simulink model "EHB_speedgoat_R2020a_V1"  (R2020a)
settings: Solver=FixedStepDiscrete  StartTime=0.0  StopTime=inf  FixedStep=0.001  RelTol=1e-3  EnableMultiTasking=on
model workspace (MAT data in the model file):
  A : Simulink.Signal (value not decoded)
  B : Simulink.Signal (value not decoded)
  C : Simulink.Signal (value not decoded)
  D : Simulink.Signal (value not decoded)
  E : Simulink.Signal (value not decoded)
  calin = [-9.96 -7.98 -5.98 -3.99 -1.994 0 1.995 3.992 5.99 7.98 9.97]
  calout = [-10 -8 -6 -4 -2 0 2 4 6 8 10]
symbols that are objects in the model workspace (value not decoded): C, D
undefined symbols (not defined in the file): Com1, none, ts_IO612
libraries: simulink x1436, xpcethercatlib x1223, yisutbxlib_utilities x256, xpcutilitieslib x156, hdlsllib x145, canmsglib x46, speedgoatlib_IO602_4 x11, speedgoatlib_IO611 x7, slrttcplib x4, CanManageLib x3, slrtlib x3, xpcseriallib x2
(part 11 of 30)

== system EHB_speedgoat_R2020a_V1/保留/TIF_01/YS4020_M_2/YS4020_M/FIU_CH13 ==
  FIU_SetCH2 : Inport
  "Bit Unpacking " : xpcutilitieslib/Bit Unpacking   SignExtend=on  MaskBitPatterns={[0],[1],[2],[3]}  MaskPackDataType=uint8  MaskPackDataSize=[1]  MaskUnpackDataTypes={'boolean','boolean','boolean','boolean'}  MaskUnpackDataSizes={[1],[1],[1],[1]}
      settings: SourceProductBaseCode=XP
  Bus Creator : BusCreator  Inputs=4
  Protect : Subsystem
  CH2_Out : Outport
  wires:
  Bus Creator/1 -> CH2_Out/1
  "Bit Unpacking "/4 -> Protect/4(Open_In)
  "Bit Unpacking "/3 -> Protect/3(COM_In)
  "Bit Unpacking "/2 -> Protect/2(KL31_In)
  "Bit Unpacking "/1 -> Protect/1(KL30_In)
  Protect/4(Open_Out) -> Bus Creator/4  "Open_Out"
  Protect/1(KL30_Out) -> Bus Creator/1  "KL30_Out"
  Protect/2(KL31_Out) -> Bus Creator/2  "KL31_Out"
  Protect/3(COM_Out) -> Bus Creator/3  "COM_Out"
  FIU_SetCH2/1 -> "Bit Unpacking "/1

== system EHB_speedgoat_R2020a_V1/保留/TIF_01/YS4020_M_2/YS4020_M/FIU_CH14 ==
  FIU_SetCH3 : Inport
  "Bit Unpacking " : xpcutilitieslib/Bit Unpacking   SignExtend=on  MaskBitPatterns={[0],[1],[2],[3]}  MaskPackDataType=uint8  MaskPackDataSize=[1]  MaskUnpackDataTypes={'boolean','boolean','boolean','boolean'}  MaskUnpackDataSizes={[1],[1],[1],[1]}
      settings: SourceProductBaseCode=XP
  Bus Creator : BusCreator  Inputs=4
  Protect : Subsystem
  CH3_Out : Outport
  wires:
  FIU_SetCH3/1 -> "Bit Unpacking "/1
  Protect/3(COM_Out) -> Bus Creator/3  "COM_Out"
  Protect/2(KL31_Out) -> Bus Creator/2  "KL31_Out"
  Protect/1(KL30_Out) -> Bus Creator/1  "KL30_Out"
  Protect/4(Open_Out) -> Bus Creator/4  "Open_Out"
  "Bit Unpacking "/1 -> Protect/1(KL30_In)
  "Bit Unpacking "/2 -> Protect/2(KL31_In)
  "Bit Unpacking "/3 -> Protect/3(COM_In)
  "Bit Unpacking "/4 -> Protect/4(Open_In)
  Bus Creator/1 -> CH3_Out/1

== system EHB_speedgoat_R2020a_V1/保留/TIF_01/YS4020_M_2/YS4020_M/FIU_CH15 ==
  FIU_SetCH4 : Inport
  "Bit Unpacking " : xpcutilitieslib/Bit Unpacking   SignExtend=on  MaskBitPatterns={[0],[1],[2],[3]}  MaskPackDataType=uint8  MaskPackDataSize=[1]  MaskUnpackDataTypes={'boolean','boolean','boolean','boolean'}  MaskUnpackDataSizes={[1],[1],[1],[1]}
      settings: SourceProductBaseCode=XP
  Bus Creator : BusCreator  Inputs=4
  Protect : Subsystem
  CH4_Out : Outport
  wires:
  Bus Creator/1 -> CH4_Out/1
  "Bit Unpacking "/4 -> Protect/4(Open_In)
  "Bit Unpacking "/3 -> Protect/3(COM_In)
  "Bit Unpacking "/2 -> Protect/2(KL31_In)
  "Bit Unpacking "/1 -> Protect/1(KL30_In)
  Protect/4(Open_Out) -> Bus Creator/4  "Open_Out"
  Protect/1(KL30_Out) -> Bus Creator/1  "KL30_Out"
  Protect/2(KL31_Out) -> Bus Creator/2  "KL31_Out"
  Protect/3(COM_Out) -> Bus Creator/3  "COM_Out"
  FIU_SetCH4/1 -> "Bit Unpacking "/1

== system EHB_speedgoat_R2020a_V1/保留/TIF_01/YS4020_M_2/YS4020_M/FIU_CH16 ==
  FIU_SetCH5 : Inport
  "Bit Unpacking " : xpcutilitieslib/Bit Unpacking   SignExtend=on  MaskBitPatterns={[0],[1],[2],[3]}  MaskPackDataType=uint8  MaskPackDataSize=[1]  MaskUnpackDataTypes={'boolean','boolean','boolean','boolean'}  MaskUnpackDataSizes={[1],[1],[1],[1]}
      settings: SourceProductBaseCode=XP
  Bus Creator : BusCreator  Inputs=4
  Protect : Subsystem
  CH5_Out : Outport
  wires:
  FIU_SetCH5/1 -> "Bit Unpacking "/1
  Protect/3(COM_Out) -> Bus Creator/3  "COM_Out"
  Protect/2(KL31_Out) -> Bus Creator/2  "KL31_Out"
  Protect/1(KL30_Out) -> Bus Creator/1  "KL30_Out"
  Protect/4(Open_Out) -> Bus Creator/4  "Open_Out"
  "Bit Unpacking "/1 -> Protect/1(KL30_In)
  "Bit Unpacking "/2 -> Protect/2(KL31_In)
  "Bit Unpacking "/3 -> Protect/3(COM_In)
  "Bit Unpacking "/4 -> Protect/4(Open_In)
  Bus Creator/1 -> CH5_Out/1

== system EHB_speedgoat_R2020a_V1/保留/TIF_01/YS4020_M_2/YS4020_M/FIU_CH17 ==
  FIU_SetCH6 : Inport
  "Bit Unpacking " : xpcutilitieslib/Bit Unpacking   SignExtend=on  MaskBitPatterns={[0],[1],[2],[3]}  MaskPackDataType=uint8  MaskPackDataSize=[1]  MaskUnpackDataTypes={'boolean','boolean','boolean','boolean'}  MaskUnpackDataSizes={[1],[1],[1],[1]}
      settings: SourceProductBaseCode=XP
  Bus Creator : BusCreator  Inputs=4
  Protect : Subsystem
  CH6_Out : Outport
  wires:
  Bus Creator/1 -> CH6_Out/1
  "Bit Unpacking "/4 -> Protect/4(Open_In)
  "Bit Unpacking "/3 -> Protect/3(COM_In)
  "Bit Unpacking "/2 -> Protect/2(KL31_In)
  "Bit Unpacking "/1 -> Protect/1(KL30_In)
  Protect/4(Open_Out) -> Bus Creator/4  "Open_Out"
  Protect/1(KL30_Out) -> Bus Creator/1  "KL30_Out"
  Protect/2(KL31_Out) -> Bus Creator/2  "KL31_Out"
  Protect/3(COM_Out) -> Bus Creator/3  "COM_Out"
  FIU_SetCH6/1 -> "Bit Unpacking "/1

== system EHB_speedgoat_R2020a_V1/保留/TIF_01/YS4020_M_2/YS4020_M/FIU_CH18 ==
  FIU_SetCH7 : Inport
  "Bit Unpacking " : xpcutilitieslib/Bit Unpacking   SignExtend=on  MaskBitPatterns={[0],[1],[2],[3]}  MaskPackDataType=uint8  MaskPackDataSize=[1]  MaskUnpackDataTypes={'boolean','boolean','boolean','boolean'}  MaskUnpackDataSizes={[1],[1],[1],[1]}
      settings: SourceProductBaseCode=XP
  Bus Creator : BusCreator  Inputs=4
  Protect : Subsystem
  CH7_Out : Outport
  wires:
  FIU_SetCH7/1 -> "Bit Unpacking "/1
  Protect/3(COM_Out) -> Bus Creator/3  "COM_Out"
  Protect/2(KL31_Out) -> Bus Creator/2  "KL31_Out"
  Protect/1(KL30_Out) -> Bus Creator/1  "KL30_Out"
  Protect/4(Open_Out) -> Bus Creator/4  "Open_Out"
  "Bit Unpacking "/1 -> Protect/1(KL30_In)
  "Bit Unpacking "/2 -> Protect/2(KL31_In)
  "Bit Unpacking "/3 -> Protect/3(COM_In)
  "Bit Unpacking "/4 -> Protect/4(Open_In)
  Bus Creator/1 -> CH7_Out/1

== system EHB_speedgoat_R2020a_V1/保留/TIF_01/YS4020_M_2/YS4020_M/FIU_CH19 ==
  FIU_SetCH8 : Inport
  "Bit Unpacking " : xpcutilitieslib/Bit Unpacking   SignExtend=on  MaskBitPatterns={[0],[1],[2],[3]}  MaskPackDataType=uint8  MaskPackDataSize=[1]  MaskUnpackDataTypes={'boolean','boolean','boolean','boolean'}  MaskUnpackDataSizes={[1],[1],[1],[1]}
      settings: SourceProductBaseCode=XP
  Bus Creator : BusCreator  Inputs=4
  Protect : Subsystem
  CH8_Out : Outport
  wires:
  Bus Creator/1 -> CH8_Out/1
  "Bit Unpacking "/4 -> Protect/4(Open_In)
  "Bit Unpacking "/3 -> Protect/3(COM_In)
  "Bit Unpacking "/2 -> Protect/2(KL31_In)
  "Bit Unpacking "/1 -> Protect/1(KL30_In)
  Protect/4(Open_Out) -> Bus Creator/4  "Open_Out"
  Protect/1(KL30_Out) -> Bus Creator/1  "KL30_Out"
  Protect/2(KL31_Out) -> Bus Creator/2  "KL31_Out"
  Protect/3(COM_Out) -> Bus Creator/3  "COM_Out"
  FIU_SetCH8/1 -> "Bit Unpacking "/1

== system EHB_speedgoat_R2020a_V1/保留/TIF_01/YS4020_M_2/YS4020_M/FIU_CH2 ==
  FIU_SetCH2 : Inport
  "Bit Unpacking " : xpcutilitieslib/Bit Unpacking   SignExtend=on  MaskBitPatterns={[0],[1],[2],[3]}  MaskPackDataType=uint8  MaskPackDataSize=[1]  MaskUnpackDataTypes={'boolean','boolean','boolean','boolean'}  MaskUnpackDataSizes={[1],[1],[1],[1]}
      settings: SourceProductBaseCode=XP
  Bus Creator : BusCreator  Inputs=4
  Protect : Subsystem
  CH2_Out : Outport
  wires:
  FIU_SetCH2/1 -> "Bit Unpacking "/1
  Protect/3(COM_Out) -> Bus Creator/3  "COM_Out"
  Protect/2(KL31_Out) -> Bus Creator/2  "KL31_Out"
  Protect/1(KL30_Out) -> Bus Creator/1  "KL30_Out"
  Protect/4(Open_Out) -> Bus Creator/4  "Open_Out"
  "Bit Unpacking "/1 -> Protect/1(KL30_In)
  "Bit Unpacking "/2 -> Protect/2(KL31_In)
  "Bit Unpacking "/3 -> Protect/3(COM_In)
  "Bit Unpacking "/4 -> Protect/4(Open_In)
  Bus Creator/1 -> CH2_Out/1

== system EHB_speedgoat_R2020a_V1/保留/TIF_01/YS4020_M_2/YS4020_M/FIU_CH20 ==
  FIU_SetCH9 : Inport
  "Bit Unpacking " : xpcutilitieslib/Bit Unpacking   SignExtend=on  MaskBitPatterns={[0],[1],[2],[3]}  MaskPackDataType=uint8  MaskPackDataSize=[1]  MaskUnpackDataTypes={'boolean','boolean','boolean','boolean'}  MaskUnpackDataSizes={[1],[1],[1],[1]}
      settings: SourceProductBaseCode=XP
  Bus Creator : BusCreator  Inputs=4
  Protect : Subsystem
  CH9_Out : Outport
  wires:
  FIU_SetCH9/1 -> "Bit Unpacking "/1
  Protect/3(COM_Out) -> Bus Creator/3  "COM_Out"
  Protect/2(KL31_Out) -> Bus Creator/2  "KL31_Out"
  Protect/1(KL30_Out) -> Bus Creator/1  "KL30_Out"
  Protect/4(Open_Out) -> Bus Creator/4  "Open_Out"
  "Bit Unpacking "/1 -> Protect/1(KL30_In)
  "Bit Unpacking "/2 -> Protect/2(KL31_In)
  "Bit Unpacking "/3 -> Protect/3(COM_In)
  "Bit Unpacking "/4 -> Protect/4(Open_In)
  Bus Creator/1 -> CH9_Out/1

== system EHB_speedgoat_R2020a_V1/保留/TIF_01/YS4020_M_2/YS4020_M/FIU_CH3 ==
  FIU_SetCH3 : Inport
  "Bit Unpacking " : xpcutilitieslib/Bit Unpacking   SignExtend=on  MaskBitPatterns={[0],[1],[2],[3]}  MaskPackDataType=uint8  MaskPackDataSize=[1]  MaskUnpackDataTypes={'boolean','boolean','boolean','boolean'}  MaskUnpackDataSizes={[1],[1],[1],[1]}
      settings: SourceProductBaseCode=XP
  Bus Creator : BusCreator  Inputs=4
  Protect : Subsystem
  CH3_Out : Outport
  wires:
  Bus Creator/1 -> CH3_Out/1
  "Bit Unpacking "/4 -> Protect/4(Open_In)
  "Bit Unpacking "/3 -> Protect/3(COM_In)
  "Bit Unpacking "/2 -> Protect/2(KL31_In)
  "Bit Unpacking "/1 -> Protect/1(KL30_In)
  Protect/4(Open_Out) -> Bus Creator/4  "Open_Out"
  Protect/1(KL30_Out) -> Bus Creator/1  "KL30_Out"
  Protect/2(KL31_Out) -> Bus Creator/2  "KL31_Out"
  Protect/3(COM_Out) -> Bus Creator/3  "COM_Out"
  FIU_SetCH3/1 -> "Bit Unpacking "/1

== system EHB_speedgoat_R2020a_V1/保留/TIF_01/YS4020_M_2/YS4020_M/FIU_CH4 ==
  FIU_SetCH4 : Inport
  "Bit Unpacking " : xpcutilitieslib/Bit Unpacking   SignExtend=on  MaskBitPatterns={[0],[1],[2],[3]}  MaskPackDataType=uint8  MaskPackDataSize=[1]  MaskUnpackDataTypes={'boolean','boolean','boolean','boolean'}  MaskUnpackDataSizes={[1],[1],[1],[1]}
      settings: SourceProductBaseCode=XP
  Bus Creator : BusCreator  Inputs=4
  Protect : Subsystem
  CH4_Out : Outport
  wires:
  FIU_SetCH4/1 -> "Bit Unpacking "/1
  Protect/3(COM_Out) -> Bus Creator/3  "COM_Out"
  Protect/2(KL31_Out) -> Bus Creator/2  "KL31_Out"
  Protect/1(KL30_Out) -> Bus Creator/1  "KL30_Out"
  Protect/4(Open_Out) -> Bus Creator/4  "Open_Out"
  "Bit Unpacking "/1 -> Protect/1(KL30_In)
  "Bit Unpacking "/2 -> Protect/2(KL31_In)
  "Bit Unpacking "/3 -> Protect/3(COM_In)
  "Bit Unpacking "/4 -> Protect/4(Open_In)
  Bus Creator/1 -> CH4_Out/1

== system EHB_speedgoat_R2020a_V1/保留/TIF_01/YS4020_M_2/YS4020_M/FIU_CH5 ==
  FIU_SetCH5 : Inport
  "Bit Unpacking " : xpcutilitieslib/Bit Unpacking   SignExtend=on  MaskBitPatterns={[0],[1],[2],[3]}  MaskPackDataType=uint8  MaskPackDataSize=[1]  MaskUnpackDataTypes={'boolean','boolean','boolean','boolean'}  MaskUnpackDataSizes={[1],[1],[1],[1]}
      settings: SourceProductBaseCode=XP
  Bus Creator : BusCreator  Inputs=4
  Protect : Subsystem
  CH5_Out : Outport
  wires:
  Bus Creator/1 -> CH5_Out/1
  "Bit Unpacking "/4 -> Protect/4(Open_In)
  "Bit Unpacking "/3 -> Protect/3(COM_In)
  "Bit Unpacking "/2 -> Protect/2(KL31_In)
  "Bit Unpacking "/1 -> Protect/1(KL30_In)
  Protect/4(Open_Out) -> Bus Creator/4  "Open_Out"
  Protect/1(KL30_Out) -> Bus Creator/1  "KL30_Out"
  Protect/2(KL31_Out) -> Bus Creator/2  "KL31_Out"
  Protect/3(COM_Out) -> Bus Creator/3  "COM_Out"
  FIU_SetCH5/1 -> "Bit Unpacking "/1

== system EHB_speedgoat_R2020a_V1/保留/TIF_01/YS4020_M_2/YS4020_M/FIU_CH6 ==
  FIU_SetCH6 : Inport
  "Bit Unpacking " : xpcutilitieslib/Bit Unpacking   SignExtend=on  MaskBitPatterns={[0],[1],[2],[3]}  MaskPackDataType=uint8  MaskPackDataSize=[1]  MaskUnpackDataTypes={'boolean','boolean','boolean','boolean'}  MaskUnpackDataSizes={[1],[1],[1],[1]}
      settings: SourceProductBaseCode=XP
  Bus Creator : BusCreator  Inputs=4
  Protect : Subsystem
  CH6_Out : Outport
  wires:
  FIU_SetCH6/1 -> "Bit Unpacking "/1
  Protect/3(COM_Out) -> Bus Creator/3  "COM_Out"
  Protect/2(KL31_Out) -> Bus Creator/2  "KL31_Out"
  Protect/1(KL30_Out) -> Bus Creator/1  "KL30_Out"
  Protect/4(Open_Out) -> Bus Creator/4  "Open_Out"
  "Bit Unpacking "/1 -> Protect/1(KL30_In)
  "Bit Unpacking "/2 -> Protect/2(KL31_In)
  "Bit Unpacking "/3 -> Protect/3(COM_In)
  "Bit Unpacking "/4 -> Protect/4(Open_In)
  Bus Creator/1 -> CH6_Out/1

== system EHB_speedgoat_R2020a_V1/保留/TIF_01/YS4020_M_2/YS4020_M/FIU_CH7 ==
  FIU_SetCH7 : Inport
  "Bit Unpacking " : xpcutilitieslib/Bit Unpacking   SignExtend=on  MaskBitPatterns={[0],[1],[2],[3]}  MaskPackDataType=uint8  MaskPackDataSize=[1]  MaskUnpackDataTypes={'boolean','boolean','boolean','boolean'}  MaskUnpackDataSizes={[1],[1],[1],[1]}
      settings: SourceProductBaseCode=XP
  Bus Creator : BusCreator  Inputs=4
  Protect : Subsystem
  CH7_Out : Outport
  wires:
  Bus Creator/1 -> CH7_Out/1
  "Bit Unpacking "/4 -> Protect/4(Open_In)
  "Bit Unpacking "/3 -> Protect/3(COM_In)
  "Bit Unpacking "/2 -> Protect/2(KL31_In)
  "Bit Unpacking "/1 -> Protect/1(KL30_In)
  Protect/4(Open_Out) -> Bus Creator/4  "Open_Out"
  Protect/1(KL30_Out) -> Bus Creator/1  "KL30_Out"
  Protect/2(KL31_Out) -> Bus Creator/2  "KL31_Out"
  Protect/3(COM_Out) -> Bus Creator/3  "COM_Out"
  FIU_SetCH7/1 -> "Bit Unpacking "/1

== system EHB_speedgoat_R2020a_V1/保留/TIF_01/YS4020_M_2/YS4020_M/FIU_CH8 ==
  FIU_SetCH8 : Inport
  "Bit Unpacking " : xpcutilitieslib/Bit Unpacking   SignExtend=on  MaskBitPatterns={[0],[1],[2],[3]}  MaskPackDataType=uint8  MaskPackDataSize=[1]  MaskUnpackDataTypes={'boolean','boolean','boolean','boolean'}  MaskUnpackDataSizes={[1],[1],[1],[1]}
      settings: SourceProductBaseCode=XP
  Bus Creator : BusCreator  Inputs=4
  Protect : Subsystem
  CH8_Out : Outport
  wires:
  FIU_SetCH8/1 -> "Bit Unpacking "/1
  Protect/3(COM_Out) -> Bus Creator/3  "COM_Out"
  Protect/2(KL31_Out) -> Bus Creator/2  "KL31_Out"
  Protect/1(KL30_Out) -> Bus Creator/1  "KL30_Out"
  Protect/4(Open_Out) -> Bus Creator/4  "Open_Out"
  "Bit Unpacking "/1 -> Protect/1(KL30_In)
  "Bit Unpacking "/2 -> Protect/2(KL31_In)
  "Bit Unpacking "/3 -> Protect/3(COM_In)
  "Bit Unpacking "/4 -> Protect/4(Open_In)
  Bus Creator/1 -> CH8_Out/1

== system EHB_speedgoat_R2020a_V1/保留/TIF_01/YS4020_M_2/YS4020_M/FIU_CH9 ==
  FIU_SetCH9 : Inport
  "Bit Unpacking " : xpcutilitieslib/Bit Unpacking   SignExtend=on  MaskBitPatterns={[0],[1],[2],[3]}  MaskPackDataType=uint8  MaskPackDataSize=[1]  MaskUnpackDataTypes={'boolean','boolean','boolean','boolean'}  MaskUnpackDataSizes={[1],[1],[1],[1]}
      settings: SourceProductBaseCode=XP
  Bus Creator : BusCreator  Inputs=4
  Protect : Subsystem
  CH9_Out : Outport
  wires:
  Bus Creator/1 -> CH9_Out/1
  "Bit Unpacking "/4 -> Protect/4(Open_In)
  "Bit Unpacking "/3 -> Protect/3(COM_In)
  "Bit Unpacking "/2 -> Protect/2(KL31_In)
  "Bit Unpacking "/1 -> Protect/1(KL30_In)
  Protect/4(Open_Out) -> Bus Creator/4  "Open_Out"
  Protect/1(KL30_Out) -> Bus Creator/1  "KL30_Out"
  Protect/2(KL31_Out) -> Bus Creator/2  "KL31_Out"
  Protect/3(COM_Out) -> Bus Creator/3  "COM_Out"
  FIU_SetCH9/1 -> "Bit Unpacking "/1

== system EHB_speedgoat_R2020a_V1/保留/TIF_01/YS4020_M_2/YS4020_M/FIU_MsgSend ==
  YS4020_M : Inport
  Enable : EnablePort
  Bus Selector : BusSelector  OutputSignals=CH1_Out.KL30_Out,CH1_Out.KL31_Out,CH1_Out.COM_Out,CH1_Out.Open_Out,CH2_Out.KL30_Out,CH2_Out.KL31_Out,CH2_Out.COM_Out,CH2_Out.Open_Out,CH3_Out.KL30_Out,CH3_Out.KL31_Out,CH3_Out.COM_Out,CH3_Out.Open_Out,CH4_Out.KL30_Out,CH4_Out.KL31_Out,CH4_Out.COM_Out,CH4_Out.Open_Out,CH5_Out.KL30_Out,CH5_Out.KL31_Out,CH5_Out.COM_Out,CH5_Out.Open_Out,CH6_Out.KL30_Out,CH6_Out.KL31_Out,CH6_Out.COM_Out,CH6_Out.Open_Out,CH7_Out.KL30_Out,CH7_Out.KL31_Out,CH7_Out.COM_Out,CH7_Out.Open_Out,CH8_Out.KL30_Out,CH8_Out.KL31_Out,CH8_Out.COM_Out,CH8_Out.Open_Out,CH9_Out.KL30_Out,CH9_Out.KL31_Out,CH9_Out.COM_Out,CH9_Out.Open_Out,CH10_Out.KL30_Out,CH10_Out.KL31_Out,CH10_Out.COM_Out,CH10_Out.Open_Out,PassWord,YS4020_M_Slot
  CAN Pack8 : canmsglib/CAN Pack  MsgList=(none)  MsgName=FIUStsSet  MsgIDType=Standard (11-bit identifier)  MsgIdentifier=1554  MsgLength=8  Remote=off  ApplyMinMax=off  BusOutput=on  SignalInfo={ 'CH10_COM', '62', '1', 'BE', 'unsigned', 'Standard', '0', '1', '0', '0', '1'; 'CH10_KL30', '60', '1', 'BE', 'unsigned', 'Standard', '0', '1', '0', '0', '1'; 'CH10_KL31', '61', '1', 'BE', 'unsigned', 'Standard', '0', '1', '0', '0', '1'; 'CH10_Open', '63', '1', 'BE', 'unsigned', 'Standard', '0', '1', '0', '0', '1'; 'CH1_COM', '26', '1', 'BE', 'unsigned', 'Standard', '0', '1', '0', '0', '1'; 'CH1_KL30', '24', '1', 'BE', 'unsigned', 'Standard', '0', '1', '0', '0', '1'; 'CH1_KL31', '25', '1', 'BE', 'unsigned', 'Standard', '0', '1', '0', '0', '1'; 'CH1_Open', '27', '1', 'BE', 'unsigned', 'Standard', '0', '1', '0', '0', '1'; 'CH2_COM', '30', '1', 'BE', 'unsigned', 'Standard', '0', '1', '0', '0', '1'; 'CH2_KL30', '28', '1', 'BE', 'unsigned', 'Standard', '0', '1', '0', '0', '1'; 'CH2_KL31', '29', '1', 'BE', 'unsigned', 'Standard', '0', '1', '0', '0', '1'; 'CH2_Open', '31', '1', 'BE', 'unsigned', 'Standard', '0', '1', '0', '0', '1'; 'CH3_COM', '34', '1', 'BE', 'unsigned', 'Standard', '0', '1', '0', '0', '1'; 'CH3_KL30', '32', '1', 'BE', 'unsigned', 'Standard', '0', '1', '0', '0', '1'; 'CH3_KL31', '33', '1', 'BE', 'unsigned', 'Standard', '0', '1', '0', '0', '1'; 'CH3_Open', '35', '1', 'BE', 'unsigned', 'Standard', '0', '1', '0', '0', '1'; 'CH4_COM', '38', '1', 'BE', 'unsigned', 'Standard', '0', '1', '0', '0', '1'; 'CH4_KL30', '36', '1', 'BE', 'unsigned', 'Standard', '0', '1', '0', '0', '1'; 'CH4_KL31', '37', '1', 'BE', 'unsigned', 'Standard', '0', '1', '0', '0', '1'; 'CH4_Open', '39', '1', 'BE', 'unsigned', 'Standard', '0', '1', '0', '0', '1'; 'CH5_COM', '42', '1', 'BE', 'unsigned', 'Standard', '0', '1', '0', '0', '1'; 'CH5_KL30', '40', '1', 'BE', 'unsigned', 'Standard', '0', '1', '0', '0', '1'; 'CH5_KL31', '41', '1', 'BE', 'unsigned', 'Standard', '0', '1', '0', '0', '1'; 'CH5_Open', '43', '1', 'BE', 'unsigned', 'Standard', '0', '1', '0', '0', '1'; 'CH6_COM', '46', '1', 'BE', 'unsigned', 'Standard', '0', '1', '0', '0', '1'; 'CH6_KL30', '44', '1', 'BE', 'unsigned', 'Standard', '0', '1', '0', '0', '1'; 'CH6_KL31', '45', '1', 'BE', 'unsigned', 'Standard', '0', '1', '0', '0', '1'; 'CH6_Open', '47', '1', 'BE', 'unsigned', 'Standard', '0', '1', '0', '0', '1'; 'CH7_COM', '50', '1', 'BE', 'unsigned', 'Standard', '0', '1', '0', '0', '1'; 'CH7_KL30', '48', '1', 'BE', 'unsigned', 'Standard', '0', '1', '0', '0', '1'; 'CH7_KL31', '49', '1', 'BE', 'unsigned', 'Standard', '0', '1', '0', '0', '1'; 'CH7_Open', '51', '1', 'BE', 'unsigned', 'Standard', '0', '1', '0', '0', '1'; 'CH8_COM', '54', '1', 'BE', 'unsigned', 'Standard', '0', '1', '0', '0', '1'; 'CH8_KL30', '52', '1', 'BE', 'unsigned', 'Standard', '0', '1', '0', '0', '1'; 'CH8_KL31', '53', '1', 'BE', 'unsigned', 'Standard', '0', '1', '0', '0', '1'; 'CH8_Open', '55', '1', 'BE', 'unsigned', 'Standard', '0', '1', '0', '0', '1'; 'CH9_COM', '58', '1', 'BE', 'unsigned', 'Standard', '0', '1', '0', '0', '1'; 'CH9_KL30', '56', '1', 'BE', 'unsigned', 'Standard', '0', '1', '0', '0', '1'; 'CH9_KL31', '57', '1', 'BE', 'unsigned', 'Standard', '0', '1', '0', '0', '1'; 'CH9_Open', '59', '1', 'BE', 'unsigned', 'Standard', '0', '1', '0', '0', '1'; 'PassWord', '16', '8', 'BE', 'unsigned', 'Standard', '0', '1', '0', '0', '15'; 'Slot', '0', '4', 'BE', 'unsigned', 'Standard', '0', '1', '0', '0', '15' }
      settings: SourceProductBaseCode=ME,VN  DataFormat=manually specified signals
  CANDataPack_ToUDP : Subsystem
  Output : Outport
  wires:
  Bus Selector/42 -> [YS4020_M_Slot]  "<YS4020_M_Slot>"
  Bus Selector/41 -> [PassWord]  "<PassWord>"
  Bus Selector/40 -> [CH10_Open]  "<Open_Out>"
  Bus Selector/39 -> [CH10_COM]  "<COM_Out>"
  Bus Selector/38 -> [CH10_KL31]  "<KL31_Out>"
  Bus Selector/37 -> [CH10_KL30]  "<KL30_Out>"
  Bus Selector/36 -> [CH9_Open]  "<Open_Out>"
  Bus Selector/35 -> [CH9_COM]  "<COM_Out>"
  Bus Selector/34 -> [CH9_KL31]  "<KL31_Out>"
  Bus Selector/33 -> [CH9_KL30]  "<KL30_Out>"
  Bus Selector/32 -> [CH8_Open]  "<Open_Out>"
  Bus Selector/31 -> [CH8_COM]  "<COM_Out>"
  Bus Selector/30 -> [CH8_KL31]  "<KL31_Out>"
  Bus Selector/29 -> [CH8_KL30]  "<KL30_Out>"
  Bus Selector/28 -> [CH7_Open]  "<Open_Out>"
  Bus Selector/27 -> [CH7_COM]  "<COM_Out>"
  Bus Selector/26 -> [CH7_KL31]  "<KL31_Out>"
  Bus Selector/25 -> [CH7_KL30]  "<KL30_Out>"
  Bus Selector/24 -> [CH6_Open]  "<Open_Out>"
  Bus Selector/23 -> [CH6_COM]  "<COM_Out>"
  Bus Selector/22 -> [CH6_KL31]  "<KL31_Out>"
  Bus Selector/21 -> [CH6_KL30]  "<KL30_Out>"
  Bus Selector/20 -> [CH5_Open]  "<Open_Out>"
  Bus Selector/19 -> [CH5_COM]  "<COM_Out>"
  Bus Selector/18 -> [CH5_KL31]  "<KL31_Out>"
  Bus Selector/17 -> [CH5_KL30]  "<KL30_Out>"
  Bus Selector/16 -> [CH4_Open]  "<Open_Out>"
  Bus Selector/15 -> [CH4_COM]  "<COM_Out>"
  Bus Selector/14 -> [CH4_KL31]  "<KL31_Out>"
  Bus Selector/13 -> [CH4_KL30]  "<KL30_Out>"
  Bus Selector/12 -> [CH3_Open]  "<Open_Out>"
  Bus Selector/11 -> [CH3_COM]  "<COM_Out>"
  Bus Selector/10 -> [CH3_KL31]  "<KL31_Out>"
  Bus Selector/9 -> [CH3_KL30]  "<KL30_Out>"
  Bus Selector/8 -> [CH2_Open]  "<Open_Out>"
  Bus Selector/7 -> [CH2_COM]  "<COM_Out>"
  Bus Selector/6 -> [CH2_KL31]  "<KL31_Out>"
  Bus Selector/5 -> [CH2_KL30]  "<KL30_Out>"
  Bus Selector/4 -> [CH1_Open]  "<Open_Out>"
  Bus Selector/3 -> [CH1_COM]  "<COM_Out>"
  Bus Selector/2 -> [CH1_KL31]  "<KL31_Out>"
  Bus Selector/1 -> [CH1_KL30]  "<KL30_Out>"
  YS4020_M/1 -> Bus Selector/1
  [PassWord] -> CAN Pack8/41  "PassWord"
  [CH9_Open] -> CAN Pack8/40  "CH9_Open"
  [CH9_KL31] -> CAN Pack8/39  "CH9_KL31"
  [CH9_KL30] -> CAN Pack8/38  "CH9_KL30"
  [CH9_COM] -> CAN Pack8/37  "CH9_COM"
  [CH8_Open] -> CAN Pack8/36  "CH8_Open"
  [CH8_KL31] -> CAN Pack8/35  "CH8_KL31"
  [CH8_KL30] -> CAN Pack8/34  "CH8_KL30"
  [CH8_COM] -> CAN Pack8/33  "CH8_COM"
  [CH7_Open] -> CAN Pack8/32  "CH7_Open"
  [CH7_KL31] -> CAN Pack8/31  "CH7_KL31"
  [CH7_KL30] -> CAN Pack8/30  "CH7_KL30"
  [CH7_COM] -> CAN Pack8/29  "CH7_COM"
  [CH6_Open] -> CAN Pack8/28  "CH6_Open"
  [CH6_KL31] -> CAN Pack8/27  "CH6_KL31"
  [CH6_KL30] -> CAN Pack8/26  "CH6_KL30"
  [CH6_COM] -> CAN Pack8/25  "CH6_COM"
  [CH5_Open] -> CAN Pack8/24  "CH5_Open"
  [CH5_KL31] -> CAN Pack8/23  "CH5_KL31"
  [CH5_KL30] -> CAN Pack8/22  "CH5_KL30"
  [CH5_COM] -> CAN Pack8/21  "CH5_COM"
  [CH4_Open] -> CAN Pack8/20  "CH4_Open"
  [CH4_KL31] -> CAN Pack8/19  "CH4_KL31"
  [CH4_KL30] -> CAN Pack8/18  "CH4_KL30"
  [CH4_COM] -> CAN Pack8/17  "CH4_COM"
  [CH3_Open] -> CAN Pack8/16  "CH3_Open"
  [CH3_KL31] -> CAN Pack8/15  "CH3_KL31"
  [CH3_KL30] -> CAN Pack8/14  "CH3_KL30"
  [CH3_COM] -> CAN Pack8/13  "CH3_COM"
  [CH2_Open] -> CAN Pack8/12  "CH2_Open"
  [CH2_KL31] -> CAN Pack8/11  "CH2_KL31"
  [CH2_KL30] -> CAN Pack8/10  "CH2_KL30"
  [CH2_COM] -> CAN Pack8/9  "CH2_COM"
  [CH1_Open] -> CAN Pack8/8  "CH1_Open"
  [CH1_KL31] -> CAN Pack8/7  "CH1_KL31"
  [CH1_KL30] -> CAN Pack8/6  "CH1_KL30"
  [CH1_COM] -> CAN Pack8/5  "CH1_COM"
  [CH10_Open] -> CAN Pack8/4  "CH10_Open"
  [CH10_KL31] -> CAN Pack8/3  "CH10_KL31"
  [CH10_KL30] -> CAN Pack8/2  "CH10_KL30"
  [CH10_COM] -> CAN Pack8/1  "CH10_COM"
  [YS4020_M_Slot] -> CAN Pack8/42  "YS4020_M_Slot"
  CAN Pack8/1 -> CANDataPack_ToUDP/1(In1)
  CANDataPack_ToUDP/1(Output) -> Output/1

== system EHB_speedgoat_R2020a_V1/保留/TIF_01/YS4020_M_2/YS4020_M/FIU_MsgSend1 ==
  YS4020_M : Inport
  Enable : EnablePort
  Bus Selector : BusSelector  OutputSignals=CH1_Out.KL30_Out,CH1_Out.KL31_Out,CH1_Out.COM_Out,CH1_Out.Open_Out,CH2_Out.KL30_Out,CH2_Out.KL31_Out,CH2_Out.COM_Out,CH2_Out.Open_Out,CH3_Out.KL30_Out,CH3_Out.KL31_Out,CH3_Out.COM_Out,CH3_Out.Open_Out,CH4_Out.KL30_Out,CH4_Out.KL31_Out,CH4_Out.COM_Out,CH4_Out.Open_Out,CH5_Out.KL30_Out,CH5_Out.KL31_Out,CH5_Out.COM_Out,CH5_Out.Open_Out,CH6_Out.KL30_Out,CH6_Out.KL31_Out,CH6_Out.COM_Out,CH6_Out.Open_Out,CH7_Out.KL30_Out,CH7_Out.KL31_Out,CH7_Out.COM_Out,CH7_Out.Open_Out,CH8_Out.KL30_Out,CH8_Out.KL31_Out,CH8_Out.COM_Out,CH8_Out.Open_Out,CH9_Out.KL30_Out,CH9_Out.KL31_Out,CH9_Out.COM_Out,CH9_Out.Open_Out,CH10_Out.KL30_Out,CH10_Out.KL31_Out,CH10_Out.COM_Out,CH10_Out.Open_Out,PassWord,YS4020_M_Slot
  CAN Pack8 : canmsglib/CAN Pack  MsgList=(none)  MsgName=FIUStsSet  MsgIDType=Standard (11-bit identifier)  MsgIdentifier=1570  MsgLength=8  Remote=off  ApplyMinMax=off  BusOutput=on  SignalInfo={ 'CH10_COM', '62', '1', 'BE', 'unsigned', 'Standard', '0', '1', '0', '0', '1'; 'CH10_KL30', '60', '1', 'BE', 'unsigned', 'Standard', '0', '1', '0', '0', '1'; 'CH10_KL31', '61', '1', 'BE', 'unsigned', 'Standard', '0', '1', '0', '0', '1'; 'CH10_Open', '63', '1', 'BE', 'unsigned', 'Standard', '0', '1', '0', '0', '1'; 'CH1_COM', '26', '1', 'BE', 'unsigned', 'Standard', '0', '1', '0', '0', '1'; 'CH1_KL30', '24', '1', 'BE', 'unsigned', 'Standard', '0', '1', '0', '0', '1'; 'CH1_KL31', '25', '1', 'BE', 'unsigned', 'Standard', '0', '1', '0', '0', '1'; 'CH1_Open', '27', '1', 'BE', 'unsigned', 'Standard', '0', '1', '0', '0', '1'; 'CH2_COM', '30', '1', 'BE', 'unsigned', 'Standard', '0', '1', '0', '0', '1'; 'CH2_KL30', '28', '1', 'BE', 'unsigned', 'Standard', '0', '1', '0', '0', '1'; 'CH2_KL31', '29', '1', 'BE', 'unsigned', 'Standard', '0', '1', '0', '0', '1'; 'CH2_Open', '31', '1', 'BE', 'unsigned', 'Standard', '0', '1', '0', '0', '1'; 'CH3_COM', '34', '1', 'BE', 'unsigned', 'Standard', '0', '1', '0', '0', '1'; 'CH3_KL30', '32', '1', 'BE', 'unsigned', 'Standard', '0', '1', '0', '0', '1'; 'CH3_KL31', '33', '1', 'BE', 'unsigned', 'Standard', '0', '1', '0', '0', '1'; 'CH3_Open', '35', '1', 'BE', 'unsigned', 'Standard', '0', '1', '0', '0', '1'; 'CH4_COM', '38', '1', 'BE', 'unsigned', 'Standard', '0', '1', '0', '0', '1'; 'CH4_KL30', '36', '1', 'BE', 'unsigned', 'Standard', '0', '1', '0', '0', '1'; 'CH4_KL31', '37', '1', 'BE', 'unsigned', 'Standard', '0', '1', '0', '0', '1'; 'CH4_Open', '39', '1', 'BE', 'unsigned', 'Standard', '0', '1', '0', '0', '1'; 'CH5_COM', '42', '1', 'BE', 'unsigned', 'Standard', '0', '1', '0', '0', '1'; 'CH5_KL30', '40', '1', 'BE', 'unsigned', 'Standard', '0', '1', '0', '0', '1'; 'CH5_KL31', '41', '1', 'BE', 'unsigned', 'Standard', '0', '1', '0', '0', '1'; 'CH5_Open', '43', '1', 'BE', 'unsigned', 'Standard', '0', '1', '0', '0', '1'; 'CH6_COM', '46', '1', 'BE', 'unsigned', 'Standard', '0', '1', '0', '0', '1'; 'CH6_KL30', '44', '1', 'BE', 'unsigned', 'Standard', '0', '1', '0', '0', '1'; 'CH6_KL31', '45', '1', 'BE', 'unsigned', 'Standard', '0', '1', '0', '0', '1'; 'CH6_Open', '47', '1', 'BE', 'unsigned', 'Standard', '0', '1', '0', '0', '1'; 'CH7_COM', '50', '1', 'BE', 'unsigned', 'Standard', '0', '1', '0', '0', '1'; 'CH7_KL30', '48', '1', 'BE', 'unsigned', 'Standard', '0', '1', '0', '0', '1'; 'CH7_KL31', '49', '1', 'BE', 'unsigned', 'Standard', '0', '1', '0', '0', '1'; 'CH7_Open', '51', '1', 'BE', 'unsigned', 'Standard', '0', '1', '0', '0', '1'; 'CH8_COM', '54', '1', 'BE', 'unsigned', 'Standard', '0', '1', '0', '0', '1'; 'CH8_KL30', '52', '1', 'BE', 'unsigned', 'Standard', '0', '1', '0', '0', '1'; 'CH8_KL31', '53', '1', 'BE', 'unsigned', 'Standard', '0', '1', '0', '0', '1'; 'CH8_Open', '55', '1', 'BE', 'unsigned', 'Standard', '0', '1', '0', '0', '1'; 'CH9_COM', '58', '1', 'BE', 'unsigned', 'Standard', '0', '1', '0', '0', '1'; 'CH9_KL30', '56', '1', 'BE', 'unsigned', 'Standard', '0', '1', '0', '0', '1'; 'CH9_KL31', '57', '1', 'BE', 'unsigned', 'Standard', '0', '1', '0', '0', '1'; 'CH9_Open', '59', '1', 'BE', 'unsigned', 'Standard', '0', '1', '0', '0', '1'; 'PassWord', '16', '8', 'BE', 'unsigned', 'Standard', '0', '1', '0', '0', '15'; 'Slot', '0', '4', 'BE', 'unsigned', 'Standard', '0', '1', '0', '0', '15' }
      settings: SourceProductBaseCode=ME,VN  DataFormat=manually specified signals
  CANDataPack_ToUDP : Subsystem
  Output : Outport
  wires:
  Bus Selector/42 -> [YS4020_M_Slot]  "<YS4020_M_Slot>"
  Bus Selector/41 -> [PassWord]  "<PassWord>"
  Bus Selector/40 -> [CH10_Open]  "<Open_Out>"
  Bus Selector/39 -> [CH10_COM]  "<COM_Out>"
  Bus Selector/38 -> [CH10_KL31]  "<KL31_Out>"
  Bus Selector/37 -> [CH10_KL30]  "<KL30_Out>"
  Bus Selector/36 -> [CH9_Open]  "<Open_Out>"
  Bus Selector/35 -> [CH9_COM]  "<COM_Out>"
  Bus Selector/34 -> [CH9_KL31]  "<KL31_Out>"
  Bus Selector/33 -> [CH9_KL30]  "<KL30_Out>"
  Bus Selector/32 -> [CH8_Open]  "<Open_Out>"
  Bus Selector/31 -> [CH8_COM]  "<COM_Out>"
  Bus Selector/30 -> [CH8_KL31]  "<KL31_Out>"
  Bus Selector/29 -> [CH8_KL30]  "<KL30_Out>"
  Bus Selector/28 -> [CH7_Open]  "<Open_Out>"
  Bus Selector/27 -> [CH7_COM]  "<COM_Out>"
  Bus Selector/26 -> [CH7_KL31]  "<KL31_Out>"
  Bus Selector/25 -> [CH7_KL30]  "<KL30_Out>"
  Bus Selector/24 -> [CH6_Open]  "<Open_Out>"
  Bus Selector/23 -> [CH6_COM]  "<COM_Out>"
  Bus Selector/22 -> [CH6_KL31]  "<KL31_Out>"
  Bus Selector/21 -> [CH6_KL30]  "<KL30_Out>"
  Bus Selector/20 -> [CH5_Open]  "<Open_Out>"
  Bus Selector/19 -> [CH5_COM]  "<COM_Out>"
  Bus Selector/18 -> [CH5_KL31]  "<KL31_Out>"
  Bus Selector/17 -> [CH5_KL30]  "<KL30_Out>"
  Bus Selector/16 -> [CH4_Open]  "<Open_Out>"
  Bus Selector/15 -> [CH4_COM]  "<COM_Out>"
  Bus Selector/14 -> [CH4_KL31]  "<KL31_Out>"
  Bus Selector/13 -> [CH4_KL30]  "<KL30_Out>"
  Bus Selector/12 -> [CH3_Open]  "<Open_Out>"
  Bus Selector/11 -> [CH3_COM]  "<COM_Out>"
  Bus Selector/10 -> [CH3_KL31]  "<KL31_Out>"
  Bus Selector/9 -> [CH3_KL30]  "<KL30_Out>"
  Bus Selector/8 -> [CH2_Open]  "<Open_Out>"
  Bus Selector/7 -> [CH2_COM]  "<COM_Out>"
  Bus Selector/6 -> [CH2_KL31]  "<KL31_Out>"
  Bus Selector/5 -> [CH2_KL30]  "<KL30_Out>"
  Bus Selector/4 -> [CH1_Open]  "<Open_Out>"
  Bus Selector/3 -> [CH1_COM]  "<COM_Out>"
  Bus Selector/2 -> [CH1_KL31]  "<KL31_Out>"
  Bus Selector/1 -> [CH1_KL30]  "<KL30_Out>"
  [YS4020_M_Slot] -> CAN Pack8/42  "YS4020_M_Slot"
  [CH10_COM] -> CAN Pack8/1  "CH10_COM"
  [CH10_KL30] -> CAN Pack8/2  "CH10_KL30"
  [CH10_KL31] -> CAN Pack8/3  "CH10_KL31"
  [CH10_Open] -> CAN Pack8/4  "CH10_Open"
  [CH1_COM] -> CAN Pack8/5  "CH1_COM"
  [CH1_KL30] -> CAN Pack8/6  "CH1_KL30"
  [CH1_KL31] -> CAN Pack8/7  "CH1_KL31"
  [CH1_Open] -> CAN Pack8/8  "CH1_Open"
  [CH2_COM] -> CAN Pack8/9  "CH2_COM"
  [CH2_KL30] -> CAN Pack8/10  "CH2_KL30"
  [CH2_KL31] -> CAN Pack8/11  "CH2_KL31"
  [CH2_Open] -> CAN Pack8/12  "CH2_Open"
  [CH3_COM] -> CAN Pack8/13  "CH3_COM"
  [CH3_KL30] -> CAN Pack8/14  "CH3_KL30"
  [CH3_KL31] -> CAN Pack8/15  "CH3_KL31"
  [CH3_Open] -> CAN Pack8/16  "CH3_Open"
  [CH4_COM] -> CAN Pack8/17  "CH4_COM"
  [CH4_KL30] -> CAN Pack8/18  "CH4_KL30"
  [CH4_KL31] -> CAN Pack8/19  "CH4_KL31"
  [CH4_Open] -> CAN Pack8/20  "CH4_Open"
  [CH5_COM] -> CAN Pack8/21  "CH5_COM"
  [CH5_KL30] -> CAN Pack8/22  "CH5_KL30"
  [CH5_KL31] -> CAN Pack8/23  "CH5_KL31"
  [CH5_Open] -> CAN Pack8/24  "CH5_Open"
  [CH6_COM] -> CAN Pack8/25  "CH6_COM"
  [CH6_KL30] -> CAN Pack8/26  "CH6_KL30"
  [CH6_KL31] -> CAN Pack8/27  "CH6_KL31"
  [CH6_Open] -> CAN Pack8/28  "CH6_Open"
  [CH7_COM] -> CAN Pack8/29  "CH7_COM"
  [CH7_KL30] -> CAN Pack8/30  "CH7_KL30"
  [CH7_KL31] -> CAN Pack8/31  "CH7_KL31"
  [CH7_Open] -> CAN Pack8/32  "CH7_Open"
  [CH8_COM] -> CAN Pack8/33  "CH8_COM"
  [CH8_KL30] -> CAN Pack8/34  "CH8_KL30"
  [CH8_KL31] -> CAN Pack8/35  "CH8_KL31"
  [CH8_Open] -> CAN Pack8/36  "CH8_Open"
  [CH9_COM] -> CAN Pack8/37  "CH9_COM"
  [CH9_KL30] -> CAN Pack8/38  "CH9_KL30"
  [CH9_KL31] -> CAN Pack8/39  "CH9_KL31"
  [CH9_Open] -> CAN Pack8/40  "CH9_Open"
  [PassWord] -> CAN Pack8/41  "PassWord"
  YS4020_M/1 -> Bus Selector/1
  CANDataPack_ToUDP/1(Output) -> Output/1
  CAN Pack8/1 -> CANDataPack_ToUDP/1(In1)

== system EHB_speedgoat_R2020a_V1/保留/TIF_01/YS4020_M_2/YS4020_M/YS4020_M_Ctrl_Trigger ==
  CH1_10 : Inport
  Bitwise Operator : simulink/Logic and Bit Operations/Bitwise Operator  logicop=OR  UseBitMask=off  BitMask=bin2dec('11011001')  BitMaskRealWorld=Stored Integer
  Demux : Demux  Outputs=10
  Detect Change : simulink/Logic and Bit Operations/Detect Change  vinit=0  OutDataTypeStr=boolean
  Mux : Mux  Inputs=10
  YS4020_M_CtrlTrigger : Outport
  wires:
  Demux/10 -> Mux/10
  Demux/9 -> Mux/9
  Demux/8 -> Mux/8
  Demux/7 -> Mux/7
  Demux/6 -> Mux/6
  Demux/5 -> Mux/5
  Demux/4 -> Mux/4
  Demux/3 -> Mux/3
  Demux/2 -> Mux/2
  Demux/1 -> Mux/1
  CH1_10/1 -> Demux/1
  Bitwise Operator/1 -> YS4020_M_CtrlTrigger/1
  Mux/1 -> Detect Change/1
  Detect Change/1 -> Bitwise Operator/1

== system EHB_speedgoat_R2020a_V1/保留/TIF_01/YS4020_M_2/YS4020_M/YS4020_M_Ctrl_Trigger1 ==
  CH11_20 : Inport
  Bitwise Operator : simulink/Logic and Bit Operations/Bitwise Operator  logicop=OR  UseBitMask=off  BitMask=bin2dec('11011001')  BitMaskRealWorld=Stored Integer
  Demux1 : Demux  Outputs=10
  Detect Change : simulink/Logic and Bit Operations/Detect Change  vinit=0  OutDataTypeStr=boolean
  Mux : Mux  Inputs=10
  YS4020_M_CtrlTrigger : Outport
  wires:
  Detect Change/1 -> Bitwise Operator/1
  Mux/1 -> Detect Change/1
  Bitwise Operator/1 -> YS4020_M_CtrlTrigger/1
  Demux1/1 -> Mux/1
  Demux1/2 -> Mux/2
  Demux1/3 -> Mux/3
  Demux1/4 -> Mux/4
  Demux1/5 -> Mux/5
  Demux1/6 -> Mux/6
  Demux1/7 -> Mux/7
  Demux1/8 -> Mux/8
  Demux1/9 -> Mux/9
  Demux1/10 -> Mux/10
  CH11_20/1 -> Demux1/1

== system EHB_speedgoat_R2020a_V1/保留/TIF_03/CB1032_3/DIO/DI ==
  Bit Slice high0 : hdlsllib/Logic and Bit Operations/Bit Slice  lidx=0  ridx=0
      settings: SourceProductBaseCode=SL
  Bit Slice high1 : hdlsllib/Logic and Bit Operations/Bit Slice  lidx=1  ridx=1
      settings: SourceProductBaseCode=SL
  Bit Slice high10 : hdlsllib/Logic and Bit Operations/Bit Slice  lidx=10  ridx=10
      settings: SourceProductBaseCode=SL
  Bit Slice high11 : hdlsllib/Logic and Bit Operations/Bit Slice  lidx=11  ridx=11
      settings: SourceProductBaseCode=SL
  Bit Slice high12 : hdlsllib/Logic and Bit Operations/Bit Slice  lidx=12  ridx=12
      settings: SourceProductBaseCode=SL
  Bit Slice high13 : hdlsllib/Logic and Bit Operations/Bit Slice  lidx=13  ridx=13
      settings: SourceProductBaseCode=SL
  Bit Slice high14 : hdlsllib/Logic and Bit Operations/Bit Slice  lidx=14  ridx=14
      settings: SourceProductBaseCode=SL
  Bit Slice high15 : hdlsllib/Logic and Bit Operations/Bit Slice  lidx=15  ridx=15
      settings: SourceProductBaseCode=SL
  Bit Slice high2 : hdlsllib/Logic and Bit Operations/Bit Slice  lidx=2  ridx=2
      settings: SourceProductBaseCode=SL
  Bit Slice high3 : hdlsllib/Logic and Bit Operations/Bit Slice  lidx=3  ridx=3
      settings: SourceProductBaseCode=SL
  Bit Slice high4 : hdlsllib/Logic and Bit Operations/Bit Slice  lidx=4  ridx=4
      settings: SourceProductBaseCode=SL
  Bit Slice high5 : hdlsllib/Logic and Bit Operations/Bit Slice  lidx=5  ridx=5
      settings: SourceProductBaseCode=SL
  Bit Slice high6 : hdlsllib/Logic and Bit Operations/Bit Slice  lidx=6  ridx=6
      settings: SourceProductBaseCode=SL
  Bit Slice high7 : hdlsllib/Logic and Bit Operations/Bit Slice  lidx=7  ridx=7
      settings: SourceProductBaseCode=SL
  Bit Slice high8 : hdlsllib/Logic and Bit Operations/Bit Slice  lidx=8  ridx=8
      settings: SourceProductBaseCode=SL
  Bit Slice high9 : hdlsllib/Logic and Bit Operations/Bit Slice  lidx=9  ridx=9
      settings: SourceProductBaseCode=SL
  Bit Slice low0 : hdlsllib/Logic and Bit Operations/Bit Slice  lidx=0  ridx=0
      settings: SourceProductBaseCode=SL
  Bit Slice low1 : hdlsllib/Logic and Bit Operations/Bit Slice  lidx=1  ridx=1
      settings: SourceProductBaseCode=SL
  Bit Slice low10 : hdlsllib/Logic and Bit Operations/Bit Slice  lidx=10  ridx=10
      settings: SourceProductBaseCode=SL
  Bit Slice low11 : hdlsllib/Logic and Bit Operations/Bit Slice  lidx=11  ridx=11
      settings: SourceProductBaseCode=SL
  Bit Slice low12 : hdlsllib/Logic and Bit Operations/Bit Slice  lidx=12  ridx=12
      settings: SourceProductBaseCode=SL
  Bit Slice low13 : hdlsllib/Logic and Bit Operations/Bit Slice  lidx=13  ridx=13
      settings: SourceProductBaseCode=SL
  Bit Slice low14 : hdlsllib/Logic and Bit Operations/Bit Slice  lidx=14  ridx=14
      settings: SourceProductBaseCode=SL
  Bit Slice low15 : hdlsllib/Logic and Bit Operations/Bit Slice  lidx=15  ridx=15
      settings: SourceProductBaseCode=SL
  Bit Slice low2 : hdlsllib/Logic and Bit Operations/Bit Slice  lidx=2  ridx=2
      settings: SourceProductBaseCode=SL
  Bit Slice low3 : hdlsllib/Logic and Bit Operations/Bit Slice  lidx=3  ridx=3
      settings: SourceProductBaseCode=SL
  Bit Slice low4 : hdlsllib/Logic and Bit Operations/Bit Slice  lidx=4  ridx=4
      settings: SourceProductBaseCode=SL
  Bit Slice low5 : hdlsllib/Logic and Bit Operations/Bit Slice  lidx=5  ridx=5
      settings: SourceProductBaseCode=SL
  Bit Slice low6 : hdlsllib/Logic and Bit Operations/Bit Slice  lidx=6  ridx=6
      settings: SourceProductBaseCode=SL
  Bit Slice low7 : hdlsllib/Logic and Bit Operations/Bit Slice  lidx=7  ridx=7
      settings: SourceProductBaseCode=SL
  Bit Slice low8 : hdlsllib/Logic and Bit Operations/Bit Slice  lidx=8  ridx=8
      settings: SourceProductBaseCode=SL
  Bit Slice low9 : hdlsllib/Logic and Bit Operations/Bit Slice  lidx=9  ridx=9
      settings: SourceProductBaseCode=SL
  DI_{1..32} (32 alike) : Gain
  DTCB CH_17_32 : DataTypeConversion  OutDataTypeStr=uint16
  DTCB CH_1_16 : DataTypeConversion  OutDataTypeStr=uint16
  EtherCAT PDO Receive1 : xpcethercatlib/EtherCAT PDO Receive  Priority=2  sig_name=Box 3 (YISUWORLD_Dig).PDOGetValue process data mapping.DIL  sig_offset=5704  sig_type=uint16  type_size=16  sig_dim=1  device_id=0  sample_time=0.001000
      settings: SourceProductBaseCode=XP
  EtherCAT PDO Receive2 : xpcethercatlib/EtherCAT PDO Receive  Priority=2  sig_name=Box 3 (YISUWORLD_Dig).PDOGetValue process data mapping.DIH  sig_offset=5688  sig_type=uint16  type_size=16  sig_dim=1  device_id=0  sample_time=0.001000
      settings: SourceProductBaseCode=XP
  DI_CH1 : Outport
  DI_CH2 : Outport  Port=2
  DI_CH3 : Outport  Port=3
  DI_CH4 : Outport  Port=4
  DI_CH5 : Outport  Port=5
  DI_CH6 : Outport  Port=6
  DI_CH7 : Outport  Port=7
  DI_CH8 : Outport  Port=8
  DI_CH9 : Outport  Port=9
  DI_CH10 : Outport  Port=10
  DI_CH11 : Outport  Port=11
  DI_CH12 : Outport  Port=12
  DI_CH13 : Outport  Port=13
  DI_CH14 : Outport  Port=14
  DI_CH15 : Outport  Port=15
  DI_CH16 : Outport  Port=16
  DI_CH17 : Outport  Port=17
  DI_CH18 : Outport  Port=18
  DI_CH19 : Outport  Port=19
  DI_CH20 : Outport  Port=20
  DI_CH21 : Outport  Port=21
  DI_CH22 : Outport  Port=22
  DI_CH23 : Outport  Port=23
  DI_CH24 : Outport  Port=24
  DI_CH25 : Outport  Port=25
  DI_CH26 : Outport  Port=26
  DI_CH27 : Outport  Port=27
  DI_CH28 : Outport  Port=28
  DI_CH29 : Outport  Port=29
  DI_CH30 : Outport  Port=30
  DI_CH31 : Outport  Port=31
  DI_CH32 : Outport  Port=32
  wires:
  EtherCAT PDO Receive1/1 -> DTCB CH_1_16/1
  DTCB CH_1_16/1 -> Bit Slice low0/1, Bit Slice low1/1, Bit Slice low2/1, Bit Slice low3/1, Bit Slice low4/1, Bit Slice low5/1, Bit Slice low6/1, Bit Slice low7/1, Bit Slice low8/1, Bit Slice low9/1, Bit Slice low10/1, Bit Slice low11/1, Bit Slice low12/1, Bit Slice low13/1, Bit Slice low14/1, Bit Slice low15/1
  Bit Slice low0/1 -> DI_1/1
  DI_1/1 -> DI_CH1/1  "DI_CH1"
  Bit Slice low1/1 -> DI_2/1
  DI_2/1 -> DI_CH2/1  "DI_CH2"
  Bit Slice low2/1 -> DI_3/1
  DI_3/1 -> DI_CH3/1  "DI_CH3"
  Bit Slice low3/1 -> DI_4/1
  DI_4/1 -> DI_CH4/1  "DI_CH4"
  Bit Slice low4/1 -> DI_5/1
  DI_5/1 -> DI_CH5/1  "DI_CH5"
  Bit Slice low5/1 -> DI_6/1
  DI_6/1 -> DI_CH6/1  "DI_CH6"
  Bit Slice low6/1 -> DI_7/1
  DI_7/1 -> DI_CH7/1  "DI_CH7"
  Bit Slice low7/1 -> DI_8/1
  DI_8/1 -> DI_CH8/1  "DI_CH8"
  Bit Slice low8/1 -> DI_9/1
  DI_9/1 -> DI_CH9/1  "DI_CH9"
  Bit Slice low9/1 -> DI_10/1
  DI_10/1 -> DI_CH10/1  "DI_CH10"
  Bit Slice low10/1 -> DI_11/1
  DI_11/1 -> DI_CH11/1  "DI_CH11"
  Bit Slice low11/1 -> DI_12/1
  DI_12/1 -> DI_CH12/1  "DI_CH12"
  Bit Slice low12/1 -> DI_13/1
  DI_13/1 -> DI_CH13/1  "DI_CH13"
  Bit Slice low13/1 -> DI_14/1
  DI_14/1 -> DI_CH14/1  "DI_CH14"
  Bit Slice low14/1 -> DI_15/1
  DI_15/1 -> DI_CH15/1  "DI_CH15"
  Bit Slice low15/1 -> DI_16/1
  DI_16/1 -> DI_CH16/1  "DI_CH16"
  EtherCAT PDO Receive2/1 -> DTCB CH_17_32/1
  DTCB CH_17_32/1 -> Bit Slice high0/1, Bit Slice high1/1, Bit Slice high2/1, Bit Slice high3/1, Bit Slice high4/1, Bit Slice high5/1, Bit Slice high6/1, Bit Slice high7/1, Bit Slice high8/1, Bit Slice high9/1, Bit Slice high10/1, Bit Slice high11/1, Bit Slice high12/1, Bit Slice high13/1, Bit Slice high14/1, Bit Slice high15/1
  Bit Slice high0/1 -> DI_17/1
  DI_17/1 -> DI_CH17/1  "DI_CH17"
  Bit Slice high1/1 -> DI_18/1
  DI_18/1 -> DI_CH18/1  "DI_CH18"
  Bit Slice high2/1 -> DI_19/1
  DI_19/1 -> DI_CH19/1  "DI_CH19"
  Bit Slice high3/1 -> DI_20/1
  DI_20/1 -> DI_CH20/1  "DI_CH20"
  Bit Slice high4/1 -> DI_21/1
  DI_21/1 -> DI_CH21/1  "DI_CH21"
  Bit Slice high5/1 -> DI_22/1
  DI_22/1 -> DI_CH22/1  "DI_CH22"
  Bit Slice high6/1 -> DI_23/1
  DI_23/1 -> DI_CH23/1  "DI_CH23"
  Bit Slice high7/1 -> DI_24/1
  DI_24/1 -> DI_CH24/1  "DI_CH24"
  Bit Slice high8/1 -> DI_25/1
  DI_25/1 -> DI_CH25/1  "DI_CH25"
  Bit Slice high9/1 -> DI_26/1
  DI_26/1 -> DI_CH26/1  "DI_CH26"
  Bit Slice high10/1 -> DI_27/1
  DI_27/1 -> DI_CH27/1  "DI_CH27"
  Bit Slice high11/1 -> DI_28/1
  DI_28/1 -> DI_CH28/1  "DI_CH28"
  Bit Slice high12/1 -> DI_29/1
  DI_29/1 -> DI_CH29/1  "DI_CH29"
  Bit Slice high13/1 -> DI_30/1
  DI_30/1 -> DI_CH30/1  "DI_CH30"
  Bit Slice high14/1 -> DI_31/1
  DI_31/1 -> DI_CH31/1  "DI_CH31"
  Bit Slice high15/1 -> DI_32/1
  DI_32/1 -> DI_CH32/1  "DI_CH32"

== system EHB_speedgoat_R2020a_V1/保留/TIF_03/CB1032_3/DIO/DO ==
  DO_CH1 : Inport
  DO_CH2 : Inport  Port=2
  DO_CH3 : Inport  Port=3
  DO_CH4 : Inport  Port=4
  DO_CH5 : Inport  Port=5
  DO_CH6 : Inport  Port=6
  DO_CH7 : Inport  Port=7
  DO_CH8 : Inport  Port=8
  DO_CH9 : Inport  Port=9
  DO_CH10 : Inport  Port=10
  DO_CH11 : Inport  Port=11
  DO_CH12 : Inport  Port=12
  DO_CH13 : Inport  Port=13
  DO_CH14 : Inport  Port=14
  DO_CH15 : Inport  Port=15
  DO_CH16 : Inport  Port=16
  DO_CH17 : Inport  Port=17
  DO_CH18 : Inport  Port=18
  DO_CH19 : Inport  Port=19
  DO_CH20 : Inport  Port=20
  DO_CH21 : Inport  Port=21
  DO_CH22 : Inport  Port=22
  DO_CH23 : Inport  Port=23
  DO_CH24 : Inport  Port=24
  DO_CH25 : Inport  Port=25
  DO_CH26 : Inport  Port=26
  DO_CH27 : Inport  Port=27
  DO_CH28 : Inport  Port=28
  DO_CH29 : Inport  Port=29
  DO_CH30 : Inport  Port=30
  DO_CH31 : Inport  Port=31
  DO_CH32 : Inport  Port=32
  DTCB CH{1..32} (32 alike) : DataTypeConversion  OutDataTypeStr=boolean
  DTCB CH_17_32 : DataTypeConversion
  DTCB CH_1_16 : DataTypeConversion
  EtherCAT PDO Transmit1 : xpcethercatlib/EtherCAT PDO Transmit   Priority=3  sig_name=Box 3 (YISUWORLD_Dig).PDOSet1 process data mapping.DL  sig_offset=5608  sig_type=uint16  type_size=16  sig_dim=1  device_id=0  sample_time=0.001000
      settings: SourceProductBaseCode=XP
  EtherCAT PDO Transmit2 : xpcethercatlib/EtherCAT PDO Transmit   Priority=3  sig_name=Box 3 (YISUWORLD_Dig).PDOSet1 process data mapping.DH  sig_offset=5592  sig_type=uint16  type_size=16  sig_dim=1  device_id=0  sample_time=0.001000
      settings: SourceProductBaseCode=XP
  bit Packing CH_17_32 : xpcutilitieslib/Bit Packing   MaskBitPatterns={[0:0],[1:1],[2:2],[3:3],[4:4],[5:5],[6:6],[7:7],[8:8],[9:9],[10:10],[11:11],[12:12],[13:13],[14:14],[15:15]}  MaskPackDataType=uint16  MaskPackDataSize=[1]
      settings: SourceProductBaseCode=XP
  bit Packing CH_1_16 : xpcutilitieslib/Bit Packing   MaskBitPatterns={[0:0],[1:1],[2:2],[3:3],[4:4],[5:5],[6:6],[7:7],[8:8],[9:9],[10:10],[11:11],[12:12],[13:13],[14:14],[15:15]}  MaskPackDataType=uint16  MaskPackDataSize=[1]
      settings: SourceProductBaseCode=XP
  wires:
  DO_CH1/1 -> DTCB CH1/1
  DO_CH2/1 -> DTCB CH2/1
  DO_CH3/1 -> DTCB CH3/1
  DO_CH4/1 -> DTCB CH4/1
  DO_CH5/1 -> DTCB CH5/1
  DO_CH6/1 -> DTCB CH6/1
  DO_CH7/1 -> DTCB CH7/1
  DO_CH8/1 -> DTCB CH8/1
  DO_CH9/1 -> DTCB CH9/1
  DO_CH10/1 -> DTCB CH10/1
  DO_CH11/1 -> DTCB CH11/1
  DO_CH12/1 -> DTCB CH12/1
  DO_CH13/1 -> DTCB CH13/1
  DO_CH14/1 -> DTCB CH14/1
  DO_CH15/1 -> DTCB CH15/1
  DO_CH16/1 -> DTCB CH16/1
  DTCB CH1/1 -> bit Packing CH_1_16/1
  DTCB CH2/1 -> bit Packing CH_1_16/2
  DTCB CH3/1 -> bit Packing CH_1_16/3
  DTCB CH4/1 -> bit Packing CH_1_16/4
  DTCB CH5/1 -> bit Packing CH_1_16/5
  DTCB CH6/1 -> bit Packing CH_1_16/6
  DTCB CH7/1 -> bit Packing CH_1_16/7
  DTCB CH8/1 -> bit Packing CH_1_16/8
  DTCB CH9/1 -> bit Packing CH_1_16/9
  DTCB CH10/1 -> bit Packing CH_1_16/10
  DTCB CH11/1 -> bit Packing CH_1_16/11
  DTCB CH12/1 -> bit Packing CH_1_16/12
  DTCB CH13/1 -> bit Packing CH_1_16/13
  DTCB CH14/1 -> bit Packing CH_1_16/14
  DTCB CH15/1 -> bit Packing CH_1_16/15
  DTCB CH16/1 -> bit Packing CH_1_16/16
  bit Packing CH_1_16/1 -> DTCB CH_1_16/1
  DTCB CH_1_16/1 -> EtherCAT PDO Transmit1/1
  DO_CH17/1 -> DTCB CH17/1
  DO_CH18/1 -> DTCB CH18/1
  DO_CH19/1 -> DTCB CH19/1
  DO_CH20/1 -> DTCB CH20/1
  DO_CH21/1 -> DTCB CH21/1
  DO_CH22/1 -> DTCB CH22/1
  DO_CH23/1 -> DTCB CH23/1
  DO_CH24/1 -> DTCB CH24/1
  DO_CH25/1 -> DTCB CH25/1
  DO_CH26/1 -> DTCB CH26/1
  DO_CH27/1 -> DTCB CH27/1
  DO_CH28/1 -> DTCB CH28/1
  DO_CH29/1 -> DTCB CH29/1
  DO_CH30/1 -> DTCB CH30/1
  DO_CH31/1 -> DTCB CH31/1
  DO_CH32/1 -> DTCB CH32/1
  DTCB CH17/1 -> bit Packing CH_17_32/1
  DTCB CH18/1 -> bit Packing CH_17_32/2
  DTCB CH19/1 -> bit Packing CH_17_32/3
  DTCB CH20/1 -> bit Packing CH_17_32/4
  DTCB CH21/1 -> bit Packing CH_17_32/5
  DTCB CH22/1 -> bit Packing CH_17_32/6
  DTCB CH23/1 -> bit Packing CH_17_32/7
  DTCB CH24/1 -> bit Packing CH_17_32/8
  DTCB CH25/1 -> bit Packing CH_17_32/9
  DTCB CH26/1 -> bit Packing CH_17_32/10
  DTCB CH27/1 -> bit Packing CH_17_32/11
  DTCB CH28/1 -> bit Packing CH_17_32/12
  DTCB CH29/1 -> bit Packing CH_17_32/13
  DTCB CH30/1 -> bit Packing CH_17_32/14
  DTCB CH31/1 -> bit Packing CH_17_32/15
  DTCB CH32/1 -> bit Packing CH_17_32/16
  bit Packing CH_17_32/1 -> DTCB CH_17_32/1
  DTCB CH_17_32/1 -> EtherCAT PDO Transmit2/1
